simulink model "helicopter_outside"  (R2026a)
settings: Solver=FixedStepAuto  FixedStep=0.001
values from neighbouring files (symbols this model uses):
  acc_period_PF = fmax_PF / f_acc    [parameters.m]    (also in parameters_parametrico.m)
  amp_outlier_acc = 0    [parameters_parametrico.m]
  amp_outlier_cam = 0    [parameters_parametrico.m]
  cam_period_PF = fmax_PF / f_cam    [parameters.m]    (also in parameters_parametrico.m)
  dt_EKF = 0.001    [parameters.m]    (also in parameters_parametrico.m)
  dt_PF = 1 / fmax_PF    [parameters.m]    (also in parameters_parametrico.m)
  helicopter_params_unc = [J_alpha_unc; J_y_unc; J_z_unc; I_b_unc; m_unc; l_unc; c_alpha_unc; c_beta_unc; eps_p_unc; eps_y_unc; g_unc]    [parameters.m]    (also in parameters_parametrico.m = helicopter_params_unc_generated)
  P0_EKF = diag([ ... (first row only)    [Params_Progetto.m]    (also in Params_Progetto_master.m; parameters.m = diag([1, 1, 1, 1]); parameters_parametrico.m = diag([10, 10, 10, 10]))
  prob_outlier = 0    [parameters_parametrico.m]
  Q_EKF = diag([ ... (first row only)    [Params_Progetto.m]    (also in Params_Progetto_master.m; parameters.m = diag([1e-6, 1e-4, 1e-6, 1e-4]); parameters_parametrico.m = diag([1e-5, 1e-3, 1e-5, 1e-3]))
  Q_PF = diag([1e-6, 1e-4, 1e-6, 1e-4])    [parameters.m]    (also in parameters_parametrico.m = diag([1e-6, 1e-2, 1e-6, 1e-2]))
  R_EKF = diag([ ... (first row only)    [Params_Progetto.m]    (also in Params_Progetto_master.m; parameters.m = diag([std_dev_cam^2, std_dev_cam^2, std_dev_acc^2]); parameters_parametrico.m)
  R_PF = diag([std_dev_cam^2, std_dev_cam^2, std_dev_acc^2])    [parameters.m]    (also in parameters_parametrico.m = diag([)
  resampling_th_PF = 0.7    [parameters.m]    (also in parameters_parametrico.m)
  std_dev_acc = 0.1    [parameters.m]    (also in parameters_parametrico.m = 1)
  std_dev_cam = 0.005    [parameters.m]    (also in parameters_parametrico.m = 0.1)
  threshold_maha = 4    [parameters_parametrico.m]
  Ts_acc = 1/f_acc    (= 0.01)    [parameters.m]    (also in parameters_parametrico.m)
  Ts_cam = 1/f_cam    (= 0.02)    [parameters.m]    (also in parameters_parametrico.m)
  W0_PF = ones(1, N_PF) / N_PF    [parameters.m]    (also in parameters_parametrico.m)
  x0 = [0; 0; 0; 0]    [parameters.m]    (also in parameters_parametrico.m = [pi/6; 0.02; pi/8; -0.03])
  x0_EKF = [0; 0; 0; 0]    [Params_Progetto.m]    (also in Params_Progetto_master.m; parameters.m; parameters_parametrico.m = [pi/2; 0.2; pi/4; -0.15])
  X0_PF = zeros(4, N_PF)    [parameters.m]    (also in parameters_parametrico.m)
  y_meas0_EKF = [0; 0; 0]    [parameters.m]    (also in parameters_parametrico.m)
libraries: simulink x1
settings Model: PacingRate=100  Creator=filin  LastModifiedBy=tomma

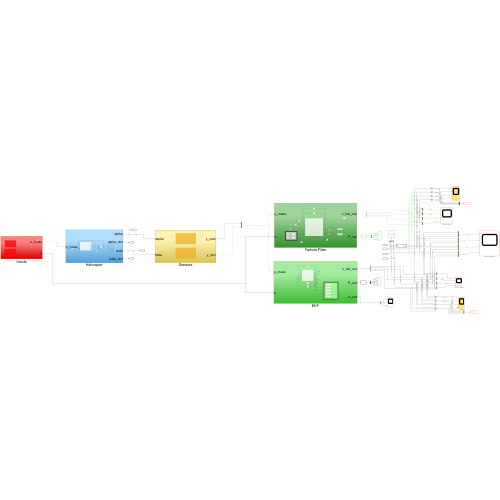
[thumbnail: Simulink's stored preview of the top-level diagram]
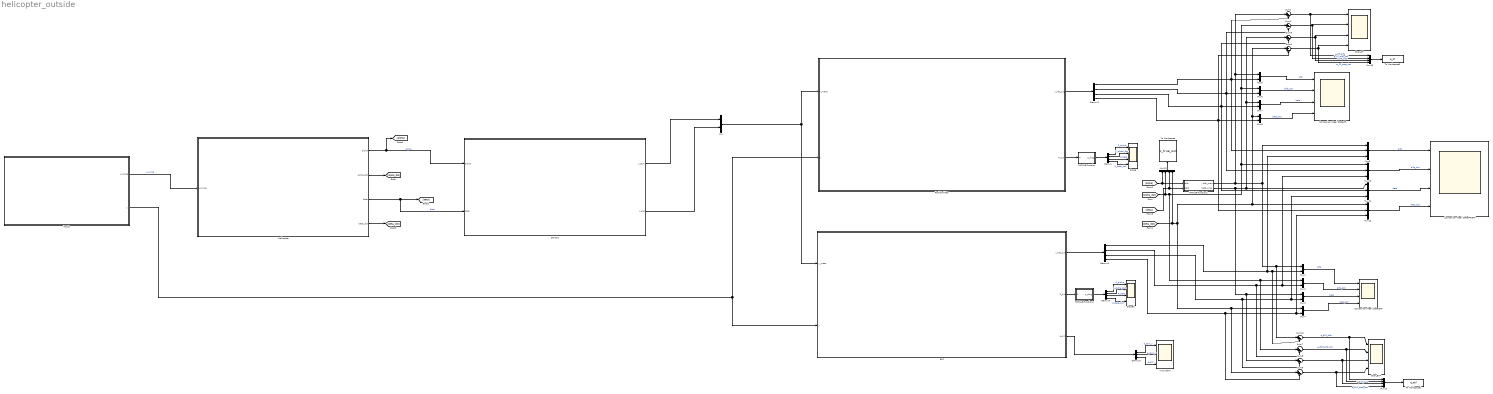
== system helicopter_outside ==
  Comparison Real State/EKF : Scope  NumInputPorts=4
      settings: ActiveDisplayYMinimum=-1.5271259237722652  ActiveDisplayYMaximum=1.3724452919901053
  Comparison Real State/PF : Scope  NumInputPorts=4
      settings: ActiveDisplayYMinimum=-1.5174521285422988  ActiveDisplayYMaximum=1.3795277031213986  DataLoggingVariableName=ScopeData2
  Comparison Real State/PF/EKF : Scope  NumInputPorts=4
      settings: ActiveDisplayYMinimum=-1.524181167386685  ActiveDisplayYMaximum=1.3704043296852875  DataLoggingVariableName=ScopeData5
  Demux{,1..2,4} (4 alike) : Demux
  Demux3 : Demux  Outputs=3
  EKF : Subsystem
  Error_EKF : Scope  NumInputPorts=4
      settings: ActiveDisplayYMinimum=-0.0192279991389335  ActiveDisplayYMaximum=0.018100458883765241  DataLoggingVariableName=ScopeData6
  Error_PF : Scope  NumInputPorts=4
      settings: ActiveDisplayYMinimum=-0.064541483866731184  ActiveDisplayYMaximum=0.058135306303903636  DataLoggingVariableName=ScopeData8
  Helicopter : Subsystem
  Innovation : Scope  NumInputPorts=3
      settings: ActiveDisplayString=3  ActiveDisplayYMinimum=-2.8043416394337108  ActiveDisplayYMaximum=8.22345062952869  DataLoggingVariableName=ScopeData4
  Inputs : Subsystem
  MATLAB Function : MATLAB Function  TreatAsAtomicUnit=on
  MATLAB Function1 : MATLAB Function  TreatAsAtomicUnit=on
  MATLAB Function2 : MATLAB Function  TreatAsAtomicUnit=on
  Mux{,1..8} (9 alike) : Mux  Inputs=2
  Mux{9..12} (4 alike) : Mux  Inputs=3
  Mux13 : Mux
  Mux14 : Mux
  Mux15 : Mux
  Particle Filter : Subsystem
  Scope : Scope  NumInputPorts=4
      settings: ActiveDisplayYMinimum=-1.6140146113413843E-5  ActiveDisplayYMaximum=0.00014720355815920033
  Scope2 : Scope  NumInputPorts=4
      settings: ActiveDisplayYMinimum=-0.12478752832079026  ActiveDisplayYMaximum=1.1234175232189243  DataLoggingVariableName=ScopeData7
  Sensors : Subsystem
  Sum{1..4,7..10} (8 alike) : Sum  Inputs=|+-
  To Workspace : ToWorkspace  VariableName=x_true_out  SampleTime=-1
  To Workspace1 : ToWorkspace  VariableName=e_ekf  SaveFormat=Timeseries  SampleTime=-1
  To Workspace2 : ToWorkspace  VariableName=e_pf  SaveFormat=Timeseries  SampleTime=-1
  wires:
  Inputs/1(u_noise) -> Helicopter/1(u_noise)  "u_noise"
  Helicopter/1(alpha) -> [alpha], Sensors/1(alpha)  "alpha"
  Helicopter/3(beta) -> [beta], Sensors/2(beta)  "beta"
  Inputs/2(u) -> Particle Filter/2(u), EKF/2(u)
  Sensors/1(y_cam) -> Mux/1
  Sensors/2(y_acc) -> Mux/2
  Mux/1 -> Particle Filter/1(y_meas), EKF/1(y_meas)
  Mux4/1 -> Comparison Real State/EKF/4  "beta_dot"
  Mux3/1 -> Comparison Real State/EKF/3  "beta"
  Mux1/1 -> Comparison Real State/EKF/1  "alfa"
  Mux2/1 -> Comparison Real State/EKF/2  "alfa_dot"
  EKF/1(x_hat_out) -> Demux1/1
  Helicopter/2(alpha_dot) -> [alpha_dot]
  Helicopter/4(beta_dot) -> [beta_dot]
  Demux1/1 -> Mux9/3, Sum10/2, Mux1/2
  Demux1/2 -> Mux10/3, Mux2/2, Sum7/2
  Demux1/3 -> Sum8/2, Mux11/3, Mux3/2
  Demux1/4 -> Mux12/3, Mux4/2, Sum9/2
  [alpha] -> Mux13/1, MATLAB Function1/1(alfa)
  [alpha_dot] -> Mux13/2, Mux10/1, Mux6/1, Sum2/1, Mux2/1, Sum7/1
  [beta_dot] -> Mux13/4, Mux12/1, Mux8/1, Sum4/1, Sum9/1, Mux4/1
  [beta] -> Mux13/3, MATLAB Function1/2(beta)
  MATLAB Function1/1(alfa_wrap) -> Sum1/1, Mux5/1, Mux9/1, Sum10/1, Mux1/1
  MATLAB Function1/2(beta_wrap) -> Mux7/1, Sum3/1, Mux11/1, Mux3/1, Sum8/1
  Particle Filter/1(x_hat_out) -> Demux2/1
  Mux6/1 -> Comparison Real State/PF/2  "alfa_dot"
  Mux7/1 -> Comparison Real State/PF/3  "beta"
  Mux5/1 -> Comparison Real State/PF/1  "alfa"
  Mux8/1 -> Comparison Real State/PF/4  "beta_dot"
  Demux2/1 -> Mux5/2, Sum1/2, Mux9/2
  Demux2/2 -> Sum2/2, Mux6/2, Mux10/2
  Demux2/3 -> Mux7/2, Sum3/2, Mux11/2
  Demux2/4 -> Mux8/2, Sum4/2, Mux12/2
  EKF/3(e_out) -> Demux3/1
  Demux3/1 -> Innovation/1  "e_cam_x"
  Demux3/3 -> Innovation/3  "e_acc"
  Demux3/2 -> Innovation/2  "e_cam_y"
  Mux11/1 -> Comparison Real State/PF/EKF/3  "beta"
  Mux10/1 -> Comparison Real State/PF/EKF/2  "alfa_dot"
  Mux9/1 -> Comparison Real State/PF/EKF/1  "alfa"
  Mux12/1 -> Comparison Real State/PF/EKF/4  "beta_dot"
  Sum9/1 -> Error_EKF/4, Mux14/4  "e_EKF_beta_dot"
  Sum10/1 -> Mux14/1, Error_EKF/1  "e_EKF_alfa"
  Sum7/1 -> Mux14/2, Error_EKF/2  "e_EKF_alfa_dot"
  Sum8/1 -> Error_EKF/3, Mux14/3  "e_EKF_beta"
  Particle Filter/2(P_out) -> MATLAB Function/1(P)
  MATLAB Function/1(p_diag) -> Demux/1
  Demux/1 -> Scope/1  "P_alpha"
  Demux/2 -> Scope/2  "P_alpha_dot"
  Demux/3 -> Scope/3  "P_beta"
  Demux/4 -> Scope/4  "P_beta_dot"
  EKF/2(P_out) -> MATLAB Function2/1(P)
  MATLAB Function2/1(p_diag) -> Demux4/1
  Demux4/4 -> Scope2/4  "P_beta_dot"
  Demux4/1 -> Scope2/1  "P_alpha"
  Demux4/2 -> Scope2/2  "P_alpha_dot"
  Demux4/3 -> Scope2/3  "P_beta"
  Mux13/1 -> To Workspace/1
  Mux14/1 -> To Workspace1/1
  Mux15/1 -> To Workspace2/1
  Sum1/1 -> Mux15/1, Error_PF/1  "e_PF_alfa"
  Sum3/1 -> Error_PF/3, Mux15/3  "e_PF_beta"
  Sum2/1 -> Mux15/2, Error_PF/2  "e_PF_alfa_dot"
  Sum4/1 -> Error_PF/4, Mux15/4  "e_PF_beta_dot"

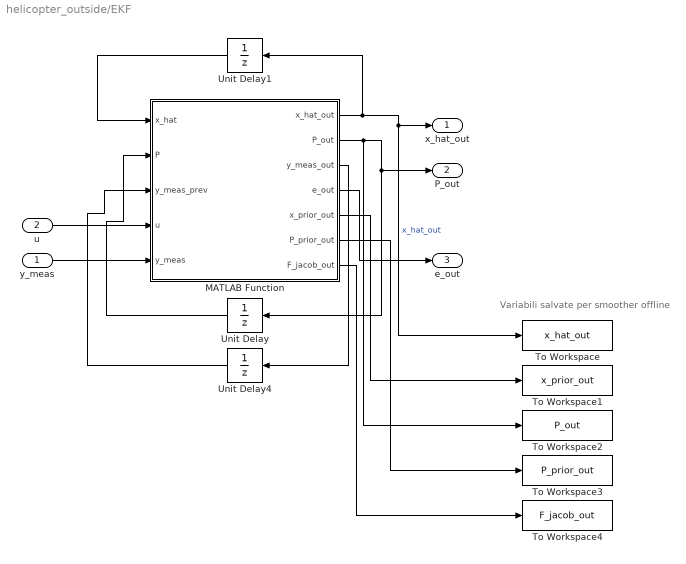
== system helicopter_outside/EKF ==
  note: Variabili salvate per smoother offline
  y_meas : Inport
  u : Inport  Port=2
  MATLAB Function : MATLAB Function  TreatAsAtomicUnit=on
  To Workspace : ToWorkspace  VariableName=x_hat_out  SampleTime=-1
  To Workspace1 : ToWorkspace  VariableName=x_prior_out  SampleTime=-1
  To Workspace2 : ToWorkspace  VariableName=P_out  SampleTime=-1
  To Workspace3 : ToWorkspace  VariableName=P_prior_out  SampleTime=-1
  To Workspace4 : ToWorkspace  VariableName=F_jacob_out  SampleTime=-1
  Unit Delay : UnitDelay  InitialCondition=P0_EKF  SampleTime=dt_EKF
  Unit Delay1 : UnitDelay  InitialCondition=x0_EKF  SampleTime=dt_EKF
  Unit Delay4 : UnitDelay  InitialCondition=y_meas0_EKF  SampleTime=dt_EKF
  x_hat_out : Outport
  P_out : Outport  Port=2
  e_out : Outport  Port=3
  wires:
  u/1 -> MATLAB Function/4(u)
  Unit Delay/1 -> MATLAB Function/2(P)
  Unit Delay1/1 -> MATLAB Function/1(x_hat)
  y_meas/1 -> MATLAB Function/5(y_meas)
  MATLAB Function/1(x_hat_out) -> To Workspace/1, x_hat_out/1, Unit Delay1/1  "x_hat_out"
  MATLAB Function/4(e_out) -> e_out/1
  MATLAB Function/2(P_out) -> To Workspace2/1, P_out/1, Unit Delay/1
  Unit Delay4/1 -> MATLAB Function/3(y_meas_prev)
  MATLAB Function/3(y_meas_out) -> Unit Delay4/1
  MATLAB Function/5(x_prior_out) -> To Workspace1/1
  MATLAB Function/6(P_prior_out) -> To Workspace3/1
  MATLAB Function/7(F_jacob_out) -> To Workspace4/1

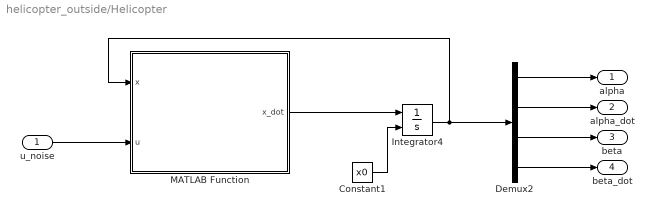
== system helicopter_outside/Helicopter ==
  u_noise : Inport
  Constant1 : Constant  Value=x0
  Demux2 : Demux
  Integrator4 : Integrator  InitialConditionSource=external
  MATLAB Function : MATLAB Function  TreatAsAtomicUnit=on
  alpha : Outport
  alpha_dot : Outport  Port=2
  beta : Outport  Port=3
  beta_dot : Outport  Port=4
  wires:
  MATLAB Function/1(x_dot) -> Integrator4/1
  Integrator4/1 -> MATLAB Function/1(x), Demux2/1
  u_noise/1 -> MATLAB Function/2(u)
  Constant1/1 -> Integrator4/2
  Demux2/1 -> alpha/1
  Demux2/2 -> alpha_dot/1
  Demux2/3 -> beta/1
  Demux2/4 -> beta_dot/1

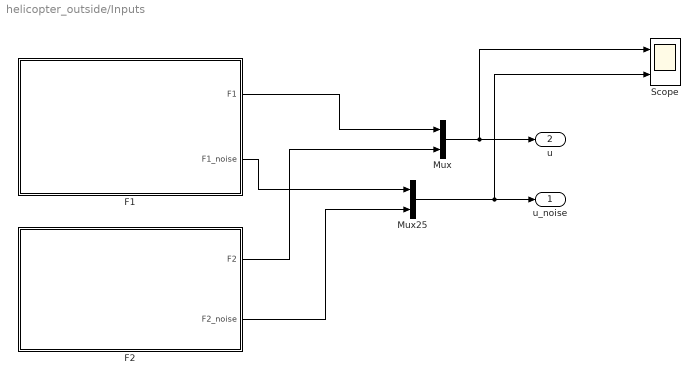
== system helicopter_outside/Inputs ==
  F1 : Subsystem
  F2 : Subsystem
  Mux : Mux  Inputs=2
  Mux25 : Mux  Inputs=2
  Scope : Scope  NumInputPorts=2
      settings: ActiveDisplayYMinimum=-1.25  ActiveDisplayYMaximum=1.25  DataLoggingVariableName=ScopeData23
  u_noise : Outport
  u : Outport  Port=2
  wires:
  Mux25/1 -> Scope/2, u_noise/1
  Mux/1 -> Scope/1, u/1
  F1/1(F1) -> Mux/1
  F1/2(F1_noise) -> Mux25/1
  F2/2(F2_noise) -> Mux25/2
  F2/1(F2) -> Mux/2

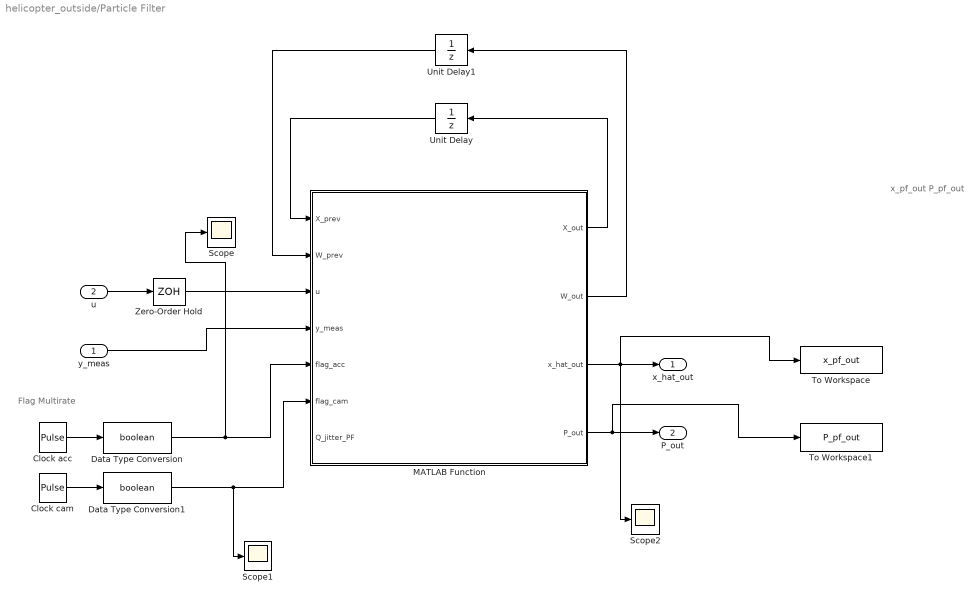
== system helicopter_outside/Particle Filter ==
  note: x_pf_out
      | P_pf_out
  note: Flag Multirate
  y_meas : Inport
  u : Inport  Port=2
  Clock acc : DiscretePulseGenerator  Period=acc_period_PF  SampleTime=dt_PF
  Clock cam : DiscretePulseGenerator  Period=cam_period_PF  SampleTime=dt_PF
  Data Type Conversion : DataTypeConversion  OutDataTypeStr=boolean  SaturateOnIntegerOverflow=off  RndMeth=Floor
  Data Type Conversion1 : DataTypeConversion  OutDataTypeStr=boolean  SaturateOnIntegerOverflow=off  RndMeth=Floor
  MATLAB Function : MATLAB Function  TreatAsAtomicUnit=on
  Scope : Scope
      settings: ActiveDisplayYMinimum=-1  ActiveDisplayYMaximum=1  DataLoggingVariableName=ScopeData11
  Scope1 : Scope
      settings: ActiveDisplayYMinimum=0.45831863800311834  ActiveDisplayYMaximum=0.46561752627326886  DataLoggingVariableName=ScopeData12
  Scope2 : Scope
      settings: ActiveDisplayYMinimum=-5.6646351318236805  ActiveDisplayYMaximum=5.4461092157236966  DataLoggingVariableName=ScopeData13
  To Workspace : ToWorkspace  VariableName=x_pf_out  SaveFormat=Timeseries  SampleTime=-1
  To Workspace1 : ToWorkspace  VariableName=P_pf_out  SaveFormat=Timeseries  SampleTime=-1
  Unit Delay : UnitDelay  InitialCondition=X0_PF  SampleTime=-1
  Unit Delay1 : UnitDelay  InitialCondition=W0_PF  SampleTime=-1
  Zero-Order Hold : ZeroOrderHold  SampleTime=dt_PF
  x_hat_out : Outport
  P_out : Outport  Port=2
  wires:
  Clock cam/1 -> Data Type Conversion1/1
  Clock acc/1 -> Data Type Conversion/1
  MATLAB Function/4(P_out) -> To Workspace1/1, P_out/1
  MATLAB Function/3(x_hat_out) -> To Workspace/1, Scope2/1, x_hat_out/1
  Data Type Conversion/1 -> Scope/1, MATLAB Function/5(flag_acc)
  Data Type Conversion1/1 -> Scope1/1, MATLAB Function/6(flag_cam)
  MATLAB Function/1(X_out) -> Unit Delay/1
  MATLAB Function/2(W_out) -> Unit Delay1/1
  Unit Delay/1 -> MATLAB Function/1(X_prev)
  Unit Delay1/1 -> MATLAB Function/2(W_prev)
  y_meas/1 -> MATLAB Function/4(y_meas)
  u/1 -> Zero-Order Hold/1
  Zero-Order Hold/1 -> MATLAB Function/3(u)

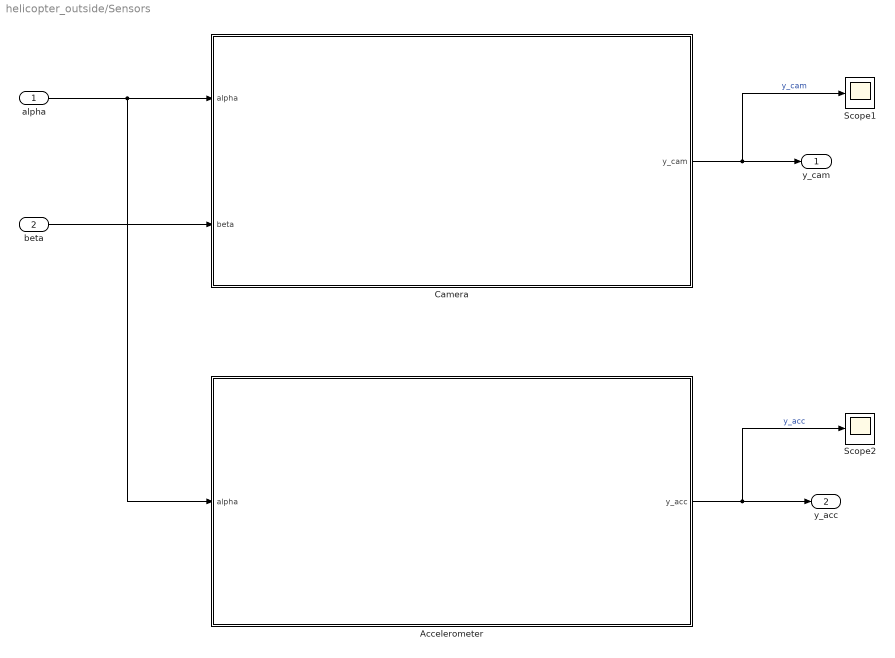
== system helicopter_outside/Sensors ==
  alpha : Inport
  beta : Inport  Port=2
  Accelerometer : Subsystem
  Camera : Subsystem
  Scope1 : Scope
      settings: ActiveDisplayYMinimum=-0.3185036970766747  ActiveDisplayYMaximum=0.83812133269721933  DataLoggingVariableName=ScopeData9
  Scope2 : Scope
      settings: ActiveDisplayYMinimum=-12.144782372783203  ActiveDisplayYMaximum=12.959158082938966  DataLoggingVariableName=ScopeData10
  y_cam : Outport
  y_acc : Outport  Port=2
  wires:
  Camera/1(y_cam) -> Scope1/1, y_cam/1  "y_cam"
  alpha/1 -> Accelerometer/1(alpha), Camera/1(alpha)
  beta/1 -> Camera/2(beta)
  Accelerometer/1(y_acc) -> Scope2/1, y_acc/1  "y_acc"

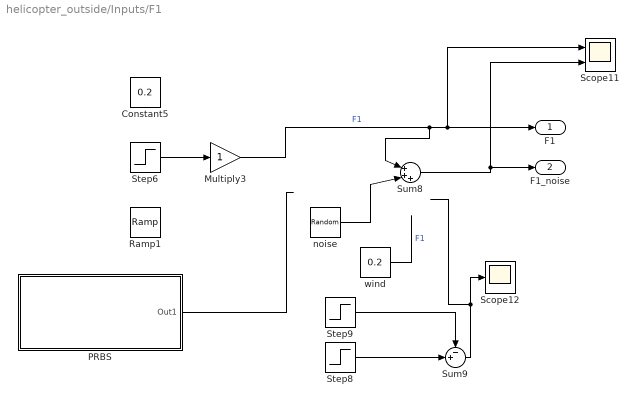
== system helicopter_outside/Inputs/F1 ==
  Constant5 : Constant  Value=0.2
  Multiply3 : Gain
  PRBS : Subsystem
  Ramp1 : simulink/Sources/Ramp  slope=0.05  start=0  InitialOutput=0
  Scope11 : Scope  NumInputPorts=2
      settings: ActiveDisplayYMinimum=-1.25  ActiveDisplayYMaximum=1.25  DataLoggingVariableName=ScopeData3
  Scope12 : Scope
      settings: ActiveDisplayYMinimum=-4.8256550057543492  ActiveDisplayYMaximum=3.2370948535299147  DataLoggingVariableName=ScopeData24
  Step6 : Step  Time=3  SampleTime=0
  Step8 : Step  Time=5  SampleTime=0
  Step9 : Step  Time=5.1  SampleTime=0
  Sum8 : Sum  Inputs=|+++
  Sum9 : Sum  Inputs=-+|
  noise : RandomNumber  Variance=0.001  Seed=5  SampleTime=0.01
  wind : Constant  Value=0.2
  F1 : Outport
  F1_noise : Outport  Port=2
  wires:
  Step9/1 -> Sum9/1
  Sum8/1 -> Scope11/2, F1_noise/1
  Multiply3/1 -> Sum8/1, Scope11/1, F1/1  "F1"
  Sum9/1 -> Scope12/1
  Step8/1 -> Sum9/2
  noise/1 -> Sum8/2
  wind/1 -> ?  "F1"
  PRBS/1(Out1) -> ?
  Step6/1 -> Multiply3/1

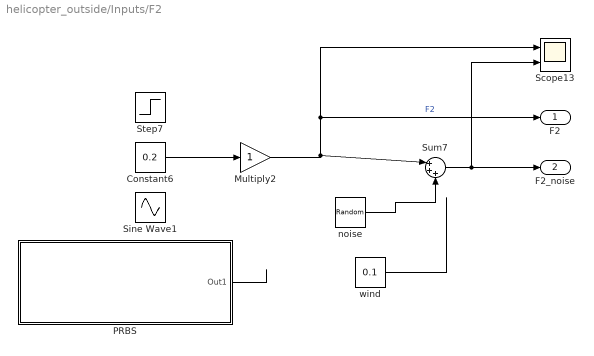
== system helicopter_outside/Inputs/F2 ==
  Constant6 : Constant  Value=0.2
  Multiply2 : Gain
  PRBS : Subsystem
  Scope13 : Scope  NumInputPorts=2
      settings: ActiveDisplayYMinimum=-1.3898816091445803  ActiveDisplayYMaximum=1.3778002922906634  DataLoggingVariableName=ScopeData25
  Sine Wave1 : Sin  Amplitude=0.5  SampleTime=0
  Step7 : Step  InitialValue=0.6  FinalValue=0.6  SampleTime=0
  Sum7 : Sum  Inputs=|+++
  noise : RandomNumber  Variance=0.001  Seed=9  SampleTime=0.01
  wind : Constant  Value=0.1
  F2 : Outport
  F2_noise : Outport  Port=2
  wires:
  Multiply2/1 -> Sum7/1, F2/1, Scope13/1  "F2"
  Constant6/1 -> Multiply2/1
  noise/1 -> Sum7/3
  Sum7/1 -> F2_noise/1, Scope13/2
  wind/1 -> ?
  PRBS/1(Out1) -> ?

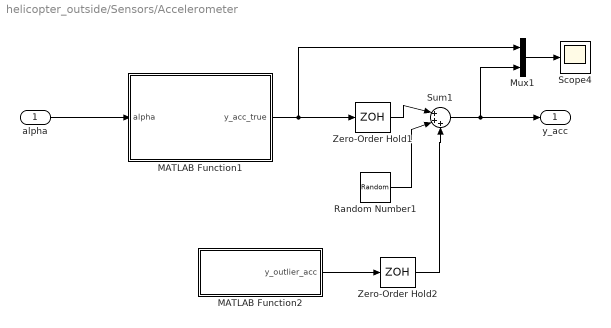
== system helicopter_outside/Sensors/Accelerometer ==
  alpha : Inport
  MATLAB Function1 : MATLAB Function  TreatAsAtomicUnit=on
  MATLAB Function2 : MATLAB Function  TreatAsAtomicUnit=on
  Mux1 : Mux  Inputs=2
  Random Number1 : RandomNumber  Variance=std_dev_acc^2  Seed=3  SampleTime=Ts_acc
  Scope4 : Scope
      settings: ActiveDisplayYMinimum=-12.144782372783203  ActiveDisplayYMaximum=12.959158082938966  DataLoggingVariableName=ScopeData4
  Sum1 : Sum  Inputs=|+++
  Zero-Order Hold1 : ZeroOrderHold  SampleTime=Ts_acc
  Zero-Order Hold2 : ZeroOrderHold  SampleTime=Ts_acc
  y_acc : Outport
  wires:
  Random Number1/1 -> Sum1/2
  Mux1/1 -> Scope4/1
  MATLAB Function1/1(y_acc_true) -> Mux1/1, Zero-Order Hold1/1
  Sum1/1 -> Mux1/2, y_acc/1
  Zero-Order Hold1/1 -> Sum1/1
  alpha/1 -> MATLAB Function1/1(alpha)
  Zero-Order Hold2/1 -> Sum1/3
  MATLAB Function2/1(y_outlier_acc) -> Zero-Order Hold2/1

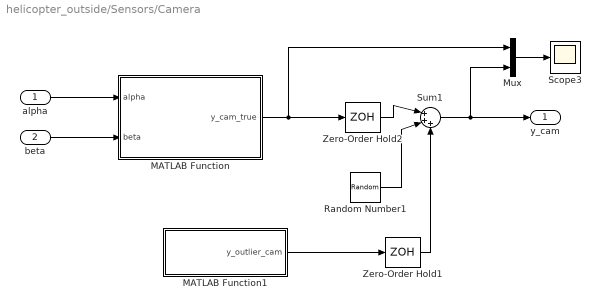
== system helicopter_outside/Sensors/Camera ==
  alpha : Inport
  beta : Inport  Port=2
  MATLAB Function : MATLAB Function  TreatAsAtomicUnit=on
  MATLAB Function1 : MATLAB Function  TreatAsAtomicUnit=on
  Mux : Mux  Inputs=2
  Random Number1 : RandomNumber  Variance=std_dev_cam^2  Seed=[1, 2]  SampleTime=Ts_cam
  Scope3 : Scope
      settings: ActiveDisplayYMinimum=-0.3185036970766747  ActiveDisplayYMaximum=0.83812133269721933  DataLoggingVariableName=ScopeData22
  Sum1 : Sum  Inputs=|+++
  Zero-Order Hold1 : ZeroOrderHold  SampleTime=Ts_cam
  Zero-Order Hold2 : ZeroOrderHold  SampleTime=Ts_cam
  y_cam : Outport
  wires:
  Sum1/1 -> Mux/2, y_cam/1
  Mux/1 -> Scope3/1
  MATLAB Function/1(y_cam_true) -> Mux/1, Zero-Order Hold2/1
  Zero-Order Hold2/1 -> Sum1/1
  Random Number1/1 -> Sum1/2
  beta/1 -> MATLAB Function/2(beta)
  alpha/1 -> MATLAB Function/1(alpha)
  MATLAB Function1/1(y_outlier_cam) -> Zero-Order Hold1/1
  Zero-Order Hold1/1 -> Sum1/3

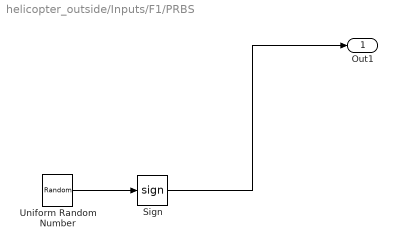
== system helicopter_outside/Inputs/F1/PRBS ==
  Sign : Signum
  Uniform Random Number : UniformRandomNumber  Minimum=-0.5  Maximum=0.5  Seed=2  SampleTime=0.1
  Out1 : Outport
  wires:
  Uniform Random Number/1 -> Sign/1
  Sign/1 -> Out1/1

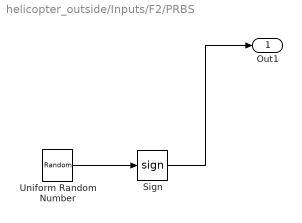
== system helicopter_outside/Inputs/F2/PRBS ==
  Sign : Signum
  Uniform Random Number : UniformRandomNumber  Minimum=-0.2  Maximum=0.2  SampleTime=0.1
  Out1 : Outport
  wires:
  Sign/1 -> Out1/1
  Uniform Random Number/1 -> Sign/1

== matlab function helicopter_outside/Particle Filter/MATLAB Function ==
  data: X_prev input size=[4, 1000]; X_out output size=[4, 1000]; W_out output size=[1, 1000]; W_prev input size=[1, 1000]; u input size=2; y_meas input size=3; flag_acc input size=1; flag_cam input size=1; x_hat_out output size=4; helicopter_params_unc parameter; Q_PF parameter; R_PF parameter; resampling_th_PF parameter; Q_jitter_PF input; P_out output size=[4, 4]; dt_PF parameter
function [X_out, W_out, x_hat_out, P_out] = PF_helicopter(X_prev, W_prev, u, y_meas, flag_acc, flag_cam, helicopter_params_unc, Q_PF, R_PF, resampling_th_PF, Q_jitter_PF, dt_PF)
    
    % PF per Elicottero 2-DOF

    % Estrazione dei comandi in ingresso
    F1 = u(1);
    F2 = u(2);
    
    % Estrazione delle misure dai sensori
    z_cam = y_meas(1:2);
    z_acc = y_meas(3);
    
    % Estrazione dei parametri fisici
    J_alpha = helicopter_params_unc(1);
    J_y     = helicopter_params_unc(2);
    J_z     = helicopter_params_unc(3);
    I_b     = helicopter_params_unc(4);
    m       = helicopter_params_unc(5);
    l       = helicopter_params_unc(6);
    c_alpha = helicopter_params_unc(7);
    c_beta  = helicopter_params_unc(8);
    eps_p   = helicopter_params_unc(9);
    eps_y   = helicopter_params_unc(10);
    g       = helicopter_params_unc(11);
    
    N = size(X_prev, 2);
    
    % Predizione
    X_pred = zeros(4, N);
    sigmas = sqrt(diag(Q_PF));
    noise = sigmas .* randn(4, N);
    
    for i = 1:N
        alpha   = X_prev(1, i);
        d_alpha = X_prev(2, i);
        beta    = X_prev(3, i);
        d_beta  = X_prev(4, i);
        
        % Equazioni di modello
        J_beta   = J_y * (sin(alpha)^2) + (J_z + m * l^2) * (cos(alpha))^2 + I_b; 
        
        dd_alpha = (- c_alpha * d_alpha - m * g * l * sin(alpha) + l * F1 * cos(beta) + eps_p * l * F2 * sin(beta)) / J_alpha;
        dd_beta  = (- c_beta * d_beta + l * F2 * cos(alpha) + eps_y * l * F1 * sin(alpha)) / J_beta;
        
        alpha_next   = wrapToPi(alpha + d_alpha * dt_PF);
        beta_next    = wrapToPi(beta + d_beta * dt_PF);
        d_alpha_next = d_alpha + dd_alpha * dt_PF;
        d_beta_next  = d_beta + dd_beta * dt_PF;
        
        X_pred(:, i) = [alpha_next; d_alpha_next; beta_next; d_beta_next];
    end
    
    % Aggiunta del rumore di processo sulle particelle predette
    X_pred = X_pred + noise;
    
    % Correzione probabilistica multirate
    W_corr = zeros(1, N); 
    inv_R_cam = inv(R_PF(1:2, 1:2));
    var_acc = R_PF(3, 3);
    
    for i = 1:N
        alpha_i = X_pred(1, i);
        beta_i  = X_pred(3, i);
        
        likelihood_acc = 1;
        likelihood_cam = 1;
        
        % Aggiornamento accelerometro
        if flag_acc
            acc_x_hat = g * sin(alpha_i);
            e_acc = z_acc - acc_x_hat;
            likelihood_acc = exp(-0.5 * (e_acc^2 / var_acc));
        end
        
        % Aggiornamento telecamera
        if flag_cam
            X_hat = l * cos(alpha_i) * cos(beta_i);
            Y_hat = l * cos(alpha_i) * sin(beta_i);
            e_cam = z_cam - [X_hat; Y_hat];
            likelihood_cam = exp(-0.5 * (e_cam' * inv_R_cam * e_cam));
        end
        
        W_corr(i) = W_prev(i) * likelihood_acc * likelihood_cam;
    end
    
    % Normalizzazione pesi
    sum_W = sum(W_corr);
    if sum_W == 0
        W_corr = ones(1, N) / N; % Gestione di sicurezza in caso di probabilità nulle
    else
        W_corr = W_corr / sum_W;
    end
    
    % Calcolo stima e varianza prima del resampling
    w = W_corr(:); 

    % Media circolare per pitch
    alpha_particelle = X_pred(1, :);
    sin_alpha_pesato = sin(alpha_particelle) * w;
    cos_alpha_pesato = cos(alpha_particelle) * w;
    alpha_media = atan2(sin_alpha_pesato, cos_alpha_pesato);
    
    % Media circolare per yaw
    beta_particelle = X_pred(3, :);
    sin_beta_pesato = sin(beta_particelle) * w;
    cos_beta_pesato = cos(beta_particelle) * w;
    beta_media = atan2(sin_beta_pesato, cos_beta_pesato);

    % Media lineare per stati non angolari
    d_alpha_media = X_pred(2, :) * w;
    d_beta_media  = X_pred(4, :) * w;
    
    x_hat_out = [alpha_media; d_alpha_media; beta_media; d_beta_media];
    
    % Varianza con correzione per la differenza angolare
    diff_stati = X_pred - x_hat_out;
    diff_stati(1,:) = wrapToPi(diff_stati(1,:)); 
    diff_stati(3,:) = wrapToPi(diff_stati(3,:)); 
    P_out = diff_stati * (W_corr .* diff_stati)';
    
    % Resampling sistematico e roughening
    X_out = zeros(4, N);
    W_out = zeros(1, N);
    indices = zeros(1, N);
    
    N_eff = 1 / sum(W_corr.^2);
    soglia_attivazione = resampling_th_PF * N;
    
    if N_eff < soglia_attivazione
        
        cumsum_W = cumsum(W_corr);
        step = 1 / N;
        u1 = rand() * step;
        
        idx = 1;
        for j = 1:N
            u_j = u1 + step * (j - 1);
            while (u_j > cumsum_W(idx)) && (idx < N)
                idx = idx + 1;
            end
            indices(j) = idx;
        end
        
        % Copia delle particelle ricampionate
        for k = 1:N
            X_out(:, k) = X_pred(:, indices(k));
        end
        
        % Aggiunta rumore artificiale post-resampling
        sigmas_jitter = sqrt(diag(Q_jitter_PF));
        jitter_noise = sigmas_jitter .* randn(4, N);
        X_out = X_out + jitter_noise;
        
        % Chiusura angolare post-jittering
        X_out(1, :) = wrapToPi(X_out(1, :)); 
        X_out(3, :) = wrapToPi(X_out(3, :)); 
        
        % Ripristino pesi uniformi
        W_out = ones(1, N) / N;
    else
        % Mantenimento particelle intatte se la soglia non è raggiunta
        X_out = X_pred;
        W_out = W_corr;
    end
end

== matlab function helicopter_outside/Sensors/Camera/MATLAB Function ==
  settings: updateMethod=DISCRETE
  data: alpha input size=1; beta input size=1; y_cam_true output size=2; helicopter_params parameter size=11
function y_cam_true = camera_sensor(alpha, beta, helicopter_params)
% Simulazione Telecamera Zenithale
% Restituisce la posizione [X; Y] ideale del marker
    
    % Estrazione parametro geometrico
    l = helicopter_params(6); % Lunghezza braccio [m]
    
    % Modello di misura h(x) ideale
    X_pos = l * cos(alpha) * cos(beta); % X marker [m]
    Y_pos = l * cos(alpha) * sin(beta); % Y marker [m]
    
    y_cam_true = [X_pos; Y_pos];
end

== matlab function helicopter_outside/Helicopter/MATLAB Function ==
  data: x input size=4; u input size=2; x_dot output size=4; helicopter_params parameter size=11
function x_dot = helicopterDynamics(x, u, helicopter_params)
% HELICOPTERDYNAMICS Calcola la derivata dello stato per l'elicottero 2-DOF
%
% Input:
%   x      : vettore di stato [alpha; alpha_dot; beta; beta_dot] (4x1)
%   u      : vettore degli ingressi [F1; F2] (2x1)
%   helicopter_params : struct contenente i parametri fisici
%
% Output:
%   x_dot  : derivata del vettore di stato (4x1)

% --- Estrazione degli stati ---
alpha     = x(1);
alpha_dot = x(2);
beta      = x(3);
beta_dot  = x(4);

% --- Estrazione degli ingressi ---
F1 = u(1);
F2 = u(2);

% Estrazione parametri dal vettore
J_alpha = helicopter_params(1);
J_y     = helicopter_params(2);
J_z     = helicopter_params(3);
I_b     = helicopter_params(4);
m       = helicopter_params(5);
l       = helicopter_params(6);
c_alpha = helicopter_params(7);
c_beta  = helicopter_params(8);
eps_p   = helicopter_params(9);
eps_y   = helicopter_params(10);
g       = helicopter_params(11);

% --- Calcolo dell'inerzia variabile ---
J_beta = J_y * sin(alpha)^2 + (J_z + m*l^2) * cos(alpha)^2 + I_b;

% --- Equazioni del moto ---
x_dot = zeros(4, 1);

x_dot(1) = alpha_dot;
x_dot(2) = (1/J_alpha) * (-c_alpha*alpha_dot - m*g*l*sin(alpha) + l*F1*cos(beta) + eps_p*l*F2*sin(beta));

x_dot(3) = beta_dot;
x_dot(4) = (1/J_beta) * (-c_beta*beta_dot + l*F2*cos(alpha) + eps_y*l*F1*sin(alpha));

end

== matlab function helicopter_outside/Sensors/Accelerometer/MATLAB Function1 ==
  settings: updateMethod=DISCRETE
  data: alpha input size=1; y_acc_true output size=1; helicopter_params parameter size=11
function y_acc_true = accelerometer_sensor(alpha, helicopter_params)
% Simulazione Accelerometro (Asse X)
% Restituisce l'accelerazione ideale letta lungo il braccio
   
    % Estrazione costante di gravità
    g = helicopter_params(11); % Accelerazione di gravità [m/s^2]
    
    % Modello di misura h(x) ideale
    y_acc_true = g * sin(alpha);
end

== matlab function helicopter_outside/EKF/MATLAB Function ==
  data: x_hat input size=4; P input size=[4, 4]; y_meas_prev input size=3; u input size=2; x_hat_out output size=4; y_meas input size=3; Q_EKF parameter; R_EKF parameter; P_out output size=[4, 4]; dt_EKF parameter; helicopter_params_unc parameter size=11; y_meas_out output size=3; e_out output size=3; threshold_maha parameter; x_prior_out output; P_prior_out output; F_jacob_out output
function [x_hat_out, P_out, y_meas_out, e_out, x_prior_out, P_prior_out, F_jacob_out] = EKF_helicopter(x_hat, P, y_meas_prev, u, y_meas, Q_EKF, R_EKF, dt_EKF, helicopter_params_unc, threshold_maha)
    
    % Assicura che gli angoli in ingresso siano compresi tra -pi e +pi
    x_hat(1) = wrapToPi(x_hat(1));
    x_hat(3) = wrapToPi(x_hat(3));
    
    % Estrazione dei parametri necessari per le equazioni di correzione
    l = helicopter_params_unc(6);
    g = helicopter_params_unc(11);
    
    % Predizione
    [x_hat_prior, P_prior, F] = predict_EKF(x_hat, P, u, helicopter_params_unc, Q_EKF, dt_EKF);
    
    % Assicura che gli angoli predetti siano compresi tra -pi e +pi
    x_hat_prior(1) = wrapToPi(x_hat_prior(1));
    x_hat_prior(3) = wrapToPi(x_hat_prior(3));
    
    % Logica multi-rate tramite rilevamento del gradino ZOH
    cam_available = any(y_meas(1:2) ~= y_meas_prev(1:2)) && all(~isnan(y_meas(1:2)));
    acc_available = (y_meas(3) ~= y_meas_prev(3)) && ~isnan(y_meas(3));
    
    % Memorizzazione delle misure correnti per il ciclo EKF successivo
    y_meas_out = y_meas;
    
    % Correzione (usa x_hat_prior come ingresso)
    if cam_available || acc_available
        [x_hat_post, P_post, e_out] = correct_EKF(x_hat_prior, P_prior, y_meas, R_EKF, l, g, cam_available, acc_available, threshold_maha);
        % ... wrapping ...
    else
        % In assenza di misure, a posteriori coincide con a priori
        x_hat_post = x_hat_prior;
        P_post = P_prior;
        e_out = zeros(3,1); 
    end
    
    % Assegnazione Finali per i Delay e per il Workspace
    x_hat_out = x_hat_post;
    P_out = P_post;
    
    x_prior_out = x_hat_prior;
    P_prior_out = P_prior;
    F_jacob_out = F;

end

function [x_hat, P, F] = predict_EKF(x_hat, P, u, params, Q_EKF, dt_EKF)
    
    % Estrazione dei parametri fisici incerti
    J_alpha = params(1); 
    J_y     = params(2); 
    J_z     = params(3); 
    I_b     = params(4);
    m       = params(5); 
    l       = params(6); 
    c_alpha = params(7); 
    c_beta  = params(8);
    eps_p   = params(9); 
    eps_y   = params(10); 
    g       = params(11);
    
    % Estrazione dei comandi
    F1 = u(1); 
    F2 = u(2);
    
    % Estrazione degli stati attuali
    a     = x_hat(1); 
    a_dot = x_hat(2); 
    b     = x_hat(3); 
    b_dot = x_hat(4);
    
    % Calcolo dell'inerzia variabile su yaw
    J_beta_val = I_b + cos(a)^2 * (J_z + l^2 * m) + J_y * sin(a)^2;
    
    % Equazioni differenziali del modello
    a_ddot = (1/J_alpha) * (-c_alpha*a_dot - m*g*l*sin(a) + l*F1*cos(b) + eps_p*l*F2*sin(b));
    b_ddot = (1/J_beta_val) * (-c_beta*b_dot + l*F2*cos(a) + eps_y*l*F1*sin(a));
    
    % Integrazione numerica di Eulero
    x_hat = x_hat + dt_EKF * [a_dot; a_ddot; b_dot; b_ddot];
    
    % Calcolo del Jacobiano del sistema
    A_c = zeros(4,4);
    A_c(1,2) = 1.0;
    A_c(2,1) = -(g * l * m * cos(a)) / J_alpha;
    A_c(2,2) = -c_alpha / J_alpha;
    A_c(2,3) = -(l * (F1 * sin(b) - F2 * eps_p * cos(b))) / J_alpha;
    A_c(3,4) = 1.0;
    A_c(4,1) = -(F2 * l * sin(a) - F1 * eps_y * l * cos(a)) / J_beta_val ...
        + (cos(a) * sin(a) * (J_z + l^2 * m) * 2.0 - J_y * cos(a) * sin(a) * 2.0) ...
        / (J_beta_val^2) * (-b_dot * c_beta + F2 * l * cos(a) + F1 * eps_y * l * sin(a));
    A_c(4,4) = -c_beta / J_beta_val;
    
    % Discretizzazione della matrice di transizione di stato
    F = eye(4) + A_c * dt_EKF;
    
    % Aggiornamento della covarianza
    P = F * P * F' + Q_EKF;
end

function [x_hat, P, e_out] = correct_EKF(x_hat, P, y_meas, R_EKF, l, g, cam_available, acc_available, threshold_maha)
    
    % Estrazione degli angoli per le matrici Jacobiane di misura
    a = x_hat(1);
    b = x_hat(3);
    
    % Flag attivazione controllo Mahalanobis
    maha_check_active = 1;
    
    % Inizializzazione dell'uscita a dimensione fissa per Simulink
    e_out = zeros(3,1);
    I_mat = eye(4);
    
    % Assemblaggio statico per singolo scenario
    if cam_available && acc_available
        
        % Entrambi i sensori disponibili
        h_x   = [l*cos(a)*cos(b); l*cos(a)*sin(b); g*sin(a)];
        H     = [-l*sin(a)*cos(b), 0, -l*cos(a)*sin(b), 0;
                 -l*sin(a)*sin(b), 0,  l*cos(a)*cos(b), 0;
                  g*cos(a),        0,  0,                0];
        y_act = [y_meas(1); y_meas(2); y_meas(3)];
        R_act = [R_EKF(1:2, 1:2), zeros(2,1); zeros(1,2), R_EKF(3,3)];
        
        e = y_act - h_x;
        S = H * P * H' + R_act;
        
        % Controllo distanza di Mahalanobis
        distance_maha = sqrt(e' / S * e);
        if distance_maha > threshold_maha && maha_check_active
            % Outlier rilevato: stato e covarianza non vengono aggiornati
        else
            L = P * H' / S; 
            x_hat = x_hat + L * e;
            P = (I_mat - L * H) * P * (I_mat - L * H)' + L * R_act * L';
        end
        
        % Assegnazione dell'innovazione all'uscita fissa
        e_out(1:3) = e;
        
    elseif cam_available && ~acc_available
        
        % Disponibile solo la telecamera
        h_x   = [l*cos(a)*cos(b); l*cos(a)*sin(b)];
        H     = [-l*sin(a)*cos(b), 0, -l*cos(a)*sin(b), 0;
                 -l*sin(a)*sin(b), 0,  l*cos(a)*cos(b), 0];
        y_act = [y_meas(1); y_meas(2)];
        R_act = R_EKF(1:2, 1:2);
        
        e = y_act - h_x;
        S = H * P * H' + R_act;
        
        % Controllo distanza di Mahalanobis
        distance_maha = sqrt(e' / S * e);
        if distance_maha > threshold_maha && maha_check_active
            % Outlier rilevato: stato e covarianza non vengono aggiornati
        else
            L = P * H' / S; 
            x_hat = x_hat + L * e;
            P = (I_mat - L * H) * P * (I_mat - L * H)' + L * R_act * L';
        end
        
        % Assegnazione parziale dell'innovazione
        e_out(1:2) = e;
        
    elseif ~cam_available && acc_available
        
        % Disponibile solo l'accelerometro
        h_x   = g*sin(a);
        H     = [g*cos(a), 0, 0, 0];
        y_act = y_meas(3);
        R_act = R_EKF(3,3);
        
        e = y_act - h_x;
        S = H * P * H' + R_act;
        
        % Controllo distanza di Mahalanobis
        distance_maha = sqrt(e' / S * e);
        if distance_maha > threshold_maha && maha_check_active
            % Outlier rilevato: stato e covarianza non vengono aggiornati
        else
            L = P * H' / S; 
            x_hat = x_hat + L * e;
            P = (I_mat - L * H) * P * (I_mat - L * H)' + L * R_act * L';
        end
        
        % Assegnazione parziale dell'innovazione
        e_out(3) = e;
    end
end

== matlab function helicopter_outside/MATLAB Function1 ==
  data: alfa input; alfa_wrap output; beta input; beta_wrap output
function [alfa_wrap, beta_wrap] = wrapper(alfa, beta)
    % Prende in ingresso il vettore di stato vero (4x1) e wrappa gli angoli
    alfa_wrap = wrapToPi(alfa);
    beta_wrap = wrapToPi(beta);
end

== matlab function helicopter_outside/MATLAB Function ==
  data: P input; p_diag output
function p_diag = extract_diag(P)
    % Estrae la diagonale principale della matrice di covarianza
    p_diag = diag(P);
end

== matlab function helicopter_outside/MATLAB Function2 ==
  data: P input; p_diag output
function p_diag = extract_diag(P)
    % Estrae la diagonale principale della matrice di covarianza
    p_diag = diag(P);
end

== matlab function helicopter_outside/Sensors/Camera/MATLAB Function1 ==
  data: y_outlier_cam output; amp_outlier_cam parameter; prob_outlier parameter
function y_outlier_cam = outlier_camera(amp_outlier_cam, prob_outlier)

    % Inizializzazione del vettore perturbazione [2x1] a zero
    y_outlier_cam = zeros(2,1);
    
    % Generazione outlier per la Telecamera (X, Y)
    if rand() < prob_outlier
        % Genera un errore casuale tra -amp_cam e +amp_cam per entrambi gli assi
        y_outlier_cam(1) = 2 * amp_outlier_cam * (rand() - 0.5);
        y_outlier_cam(2) = 2 * amp_outlier_cam * (rand() - 0.5);
    end
    
end

== matlab function helicopter_outside/Sensors/Accelerometer/MATLAB Function2 ==
  data: prob_outlier parameter; y_outlier_acc output; amp_outlier_acc parameter
function y_outlier_acc = outlier_accelerometer(prob_outlier, amp_outlier_acc)

    % Inizializzazione della perturbazione [1x1] a zero
    y_outlier_acc = 0;
    
    % Generazione outlier per l'Accelerometro (Z)
    if rand() < prob_outlier
        % Genera un errore casuale tra -amp_acc e +amp_acc
        y_outlier_acc = 2 * amp_outlier_acc * (rand() - 0.5);
    end
    
end
